simulink model "task1"  (R2022b)
settings: Solver=VariableStepAuto  StartTime=0.0  StopTime=10.0  RelTol=1e-3
values from neighbouring files (symbols this model uses):
  I = [0.07, 0.0504, 0.0109]    [task1main.m]    (also in task2main.m = diag(I); task3main.m = diag(I); task4main.m = diag(I); task5.m = [0.07; 0.0109; 0.0504])
  w0 = [0.45, 0.52, 0.55]    [task1main.m]    (also in task2main.m = [0.45; 0.52; 0.55]; task3main.m = [0.45; 0.52; 0.55]; task4main.m = cat(1,w0,wr0); task5.m = [0.01; 0.01; 2])
settings Model: Creator=a1pab  LastModifiedBy=a1pab

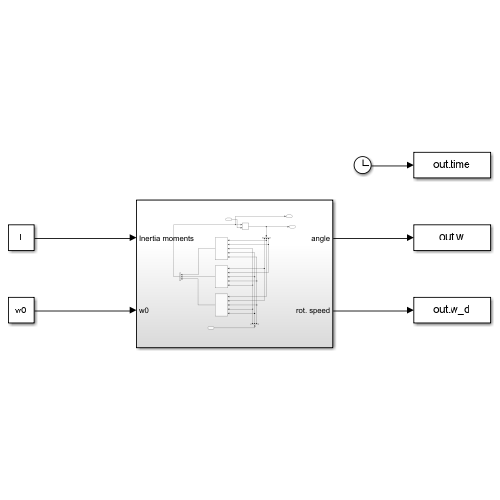
[thumbnail: Simulink's stored preview of the top-level diagram]
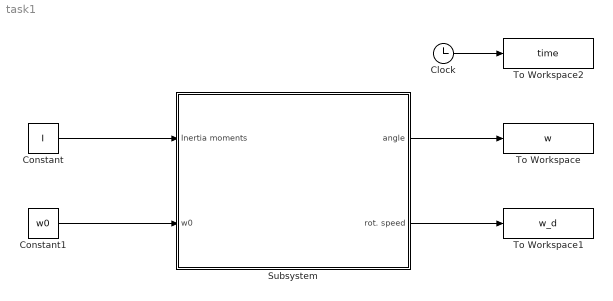
== system task1 ==
  Clock : Clock
  Constant : Constant  Value=I
  Constant1 : Constant  Value=w0
  Subsystem : Subsystem
  To Workspace : ToWorkspace  VariableName=w  SampleTime=-1
  To Workspace1 : ToWorkspace  VariableName=w_d  SampleTime=-1
  To Workspace2 : ToWorkspace  VariableName=time  SampleTime=-1
  wires:
  Subsystem/1(angle) -> To Workspace/1
  Subsystem/2(rot. speed) -> To Workspace1/1
  Constant/1 -> Subsystem/1(Inertia moments)
  Constant1/1 -> Subsystem/2(w0)
  Clock/1 -> To Workspace2/1

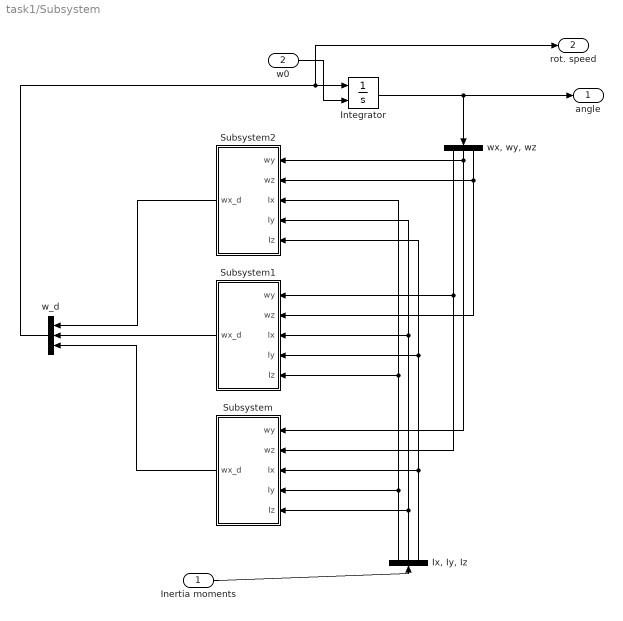
== system task1/Subsystem ==
  Inertia moments : Inport
  w0 : Inport  Port=2
  Integrator : Integrator  InitialConditionSource=external
  "Ix, Iy, Iz" : Demux  Outputs=3
  Subsystem : Subsystem
  Subsystem1 : Subsystem
  Subsystem2 : Subsystem
  w_d : Mux  Inputs=3
  "wx, wy, wz" : Demux  Outputs=3
  angle : Outport
  rot. speed : Outport  Port=2
  wires:
  Inertia moments/1 -> "Ix, Iy, Iz"/1
  w_d/1 -> rot. speed/1, Integrator/1
  Integrator/1 -> angle/1, "wx, wy, wz"/1
  w0/1 -> Integrator/2
  "wx, wy, wz"/2 -> Subsystem/1(wy), Subsystem2/1(wy)
  "wx, wy, wz"/3 -> Subsystem1/2(wz), Subsystem2/2(wz)
  "Ix, Iy, Iz"/1 -> Subsystem/4(Iy), Subsystem1/5(Iz), Subsystem2/3(Ix)
  "Ix, Iy, Iz"/2 -> Subsystem/5(Iz), Subsystem1/3(Ix), Subsystem2/4(Iy)
  "Ix, Iy, Iz"/3 -> Subsystem/3(Ix), Subsystem1/4(Iy), Subsystem2/5(Iz)
  "wx, wy, wz"/1 -> Subsystem/2(wz), Subsystem1/1(wy)
  Subsystem/1(wx_d) -> w_d/3
  Subsystem1/1(wx_d) -> w_d/2
  Subsystem2/1(wx_d) -> w_d/1

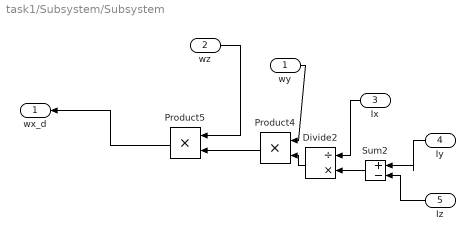
== system task1/Subsystem/Subsystem ==
  wy : Inport
  wz : Inport  Port=2
  Ix : Inport  Port=3
  Iy : Inport  Port=4
  Iz : Inport  Port=5
  Divide2 : Product  Inputs=/*
  Product4 : Product
  Product5 : Product
  Sum2 : Sum  Inputs=|+-
  wx_d : Outport
  wires:
  Divide2/1 -> Product4/2
  wy/1 -> Product4/1
  Iz/1 -> Sum2/2
  Product4/1 -> Product5/2
  Iy/1 -> Sum2/1
  Sum2/1 -> Divide2/2
  Ix/1 -> Divide2/1
  wz/1 -> Product5/1
  Product5/1 -> wx_d/1

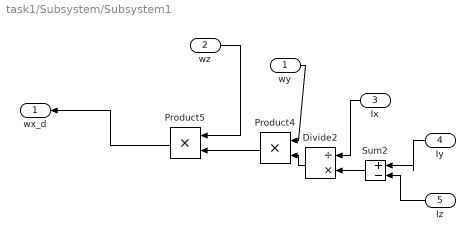
== system task1/Subsystem/Subsystem1 ==
  wy : Inport
  wz : Inport  Port=2
  Ix : Inport  Port=3
  Iy : Inport  Port=4
  Iz : Inport  Port=5
  Divide2 : Product  Inputs=/*
  Product4 : Product
  Product5 : Product
  Sum2 : Sum  Inputs=|+-
  wx_d : Outport
  wires:
  Divide2/1 -> Product4/2
  wy/1 -> Product4/1
  Iz/1 -> Sum2/2
  Product4/1 -> Product5/2
  Iy/1 -> Sum2/1
  Sum2/1 -> Divide2/2
  Ix/1 -> Divide2/1
  wz/1 -> Product5/1
  Product5/1 -> wx_d/1

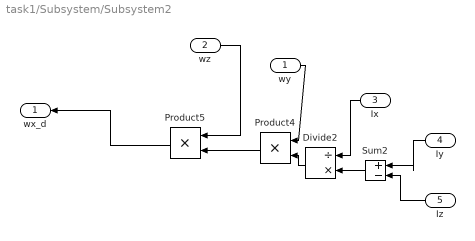
== system task1/Subsystem/Subsystem2 ==
  wy : Inport
  wz : Inport  Port=2
  Ix : Inport  Port=3
  Iy : Inport  Port=4
  Iz : Inport  Port=5
  Divide2 : Product  Inputs=/*
  Product4 : Product
  Product5 : Product
  Sum2 : Sum  Inputs=|+-
  wx_d : Outport
  wires:
  Divide2/1 -> Product4/2
  wy/1 -> Product4/1
  Iz/1 -> Sum2/2
  Product4/1 -> Product5/2
  Iy/1 -> Sum2/1
  Sum2/1 -> Divide2/2
  Ix/1 -> Divide2/1
  wz/1 -> Product5/1
  Product5/1 -> wx_d/1
